simulink model "sampleModel238_pp_991_1"  (R2021b)
settings: Solver=VariableStepAuto  StartTime=0.0  StopTime=10.0  RelTol=1e-3
undefined symbols (not defined in the file): DiscIntNeverNeededParam, Newton, Raphson
libraries: simulink x40, slpidlib x5
settings Model: Creator=user  LastModifiedBy=cemery

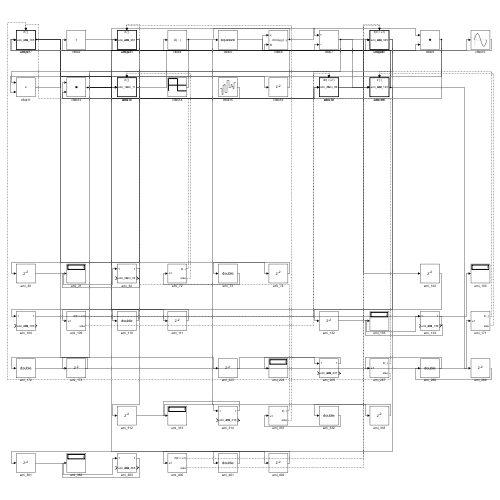
[thumbnail: Simulink's stored preview of the top-level diagram]
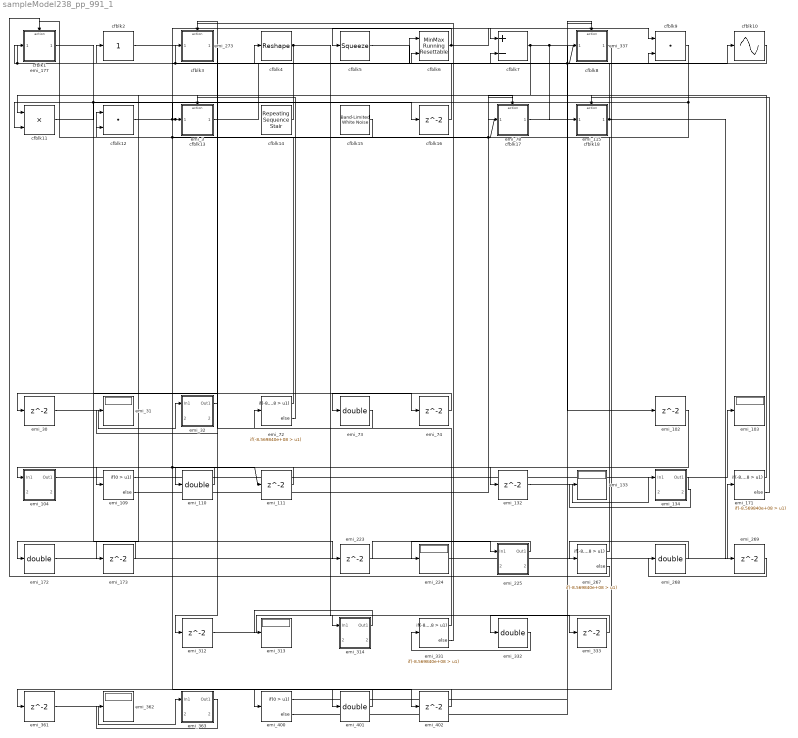
== system sampleModel238_pp_991_1 ==
  cfblk1 : Subsystem  TreatAsAtomicUnit=on
  cfblk10 : Sin  TimeSource=Use external signal  SampleTime=0
  cfblk11 : Product
  cfblk12 : DotProduct  InputSameDT=on  OutDataTypeStr=Inherit: Inherit via internal rule
  cfblk13 : Subsystem  TreatAsAtomicUnit=on
  cfblk14 : simulink/Sources/Repeating Sequence Stair  OutValues=[504987243.712228, -428491998.363153]  tsamp=-1  OutMin=[]  OutMax=[]  OutDataTypeStr=double  OutputDataTypeScalingMode=double  OutDataType=fixdt(0,8)  ConRadixGroup=Best Precision: Vector-wise  OutScaling=2^-12
  cfblk15 : simulink/Sources/Band-Limited White Noise  Cov=[8048045641.743666]  Ts=0.1  seed=[4340023928.000000]
  cfblk16 : Delay  SampleTime=1
  cfblk17 : Subsystem  TreatAsAtomicUnit=on
  cfblk18 : Subsystem  TreatAsAtomicUnit=on
  cfblk2 : simulink/Math Operations/Slider Gain  gain=1  low=0  high=2
  cfblk3 : Subsystem  TreatAsAtomicUnit=on
  cfblk4 : Reshape
  cfblk5 : Squeeze
  cfblk6 : simulink/Math Operations/MinMax Running Resettable  Function=min  vinit=0.0
  cfblk7 : Sum  Inputs=+-
  cfblk8 : Subsystem  TreatAsAtomicUnit=on
  cfblk9 : DotProduct  InputSameDT=on  OutDataTypeStr=Inherit: Inherit via internal rule
  emi_{30,102,132,361} (4 alike) : Delay  SampleTime=1
  emi_{31,103,133,224,313,362} (6 alike) : Display
  emi_104 : Subsystem
  emi_109 : If  IfExpression=0 > u1  SampleTime=1
  emi_{73,110,172,268,332,401} (6 alike) : DataTypeConversion  OutDataTypeStr=double
  emi_111 : Delay  InitialCondition=0
  emi_115 : Subsystem  TreatAsAtomicUnit=on
  emi_134 : Subsystem
  emi_171 : If  IfExpression=-8.569840e+08 > u1  SampleTime=1
  emi_{74,173,269,333} (4 alike) : Delay  InitialCondition=-428491998.3632
  emi_177 : Subsystem  TreatAsAtomicUnit=on
  emi_223 : Delay
  emi_225 : Subsystem
  emi_267 : If  IfExpression=-8.569840e+08 > u1
  emi_273 : Subsystem  TreatAsAtomicUnit=on
  emi_3 : Subsystem  TreatAsAtomicUnit=on
  emi_312 : Delay
  emi_314 : Subsystem
  emi_32 : Subsystem
  emi_331 : If  IfExpression=-8.569840e+08 > u1
  emi_337 : Subsystem  TreatAsAtomicUnit=on
  emi_363 : Subsystem
  emi_400 : If  IfExpression=0 > u1
  emi_402 : Delay  InitialCondition=0
  emi_72 : If  IfExpression=-8.569840e+08 > u1
  emi_78 : Subsystem  TreatAsAtomicUnit=on
  wires:
  cfblk14/1 -> cfblk4/1
  cfblk9/1 -> cfblk12/1, cfblk11/2
  cfblk15/1 -> cfblk12/2
  cfblk10/1 -> cfblk6/2
  cfblk2/1 -> cfblk7/1
  cfblk6/1 -> cfblk9/1, cfblk5/1
  cfblk12/1 -> emi_111/1, emi_402/1, cfblk17/1(emi_76), emi_78/1(emi_85), cfblk8/1(emi_335), emi_337/1(emi_344)
  cfblk5/1 -> cfblk7/2
  cfblk11/1 -> cfblk16/1
  cfblk16/1 -> cfblk6/1
  cfblk13/1(emi_2) -> cfblk10/1
  emi_3/1(emi_11) -> emi_30/1
  emi_30/1 -> emi_32/1(In1)
  emi_32/1(Out1) -> emi_31/1
  emi_72/2 -> cfblk13/Action
  emi_72/1 -> emi_3/Action
  emi_73/1 -> emi_72/1
  emi_74/1 -> emi_73/1
  cfblk17/1(emi_77) -> cfblk9/2
  emi_78/1(emi_86) -> emi_102/1
  emi_102/1 -> emi_104/1(In1)
  emi_104/1(Out1) -> emi_103/1
  emi_109/2 -> cfblk17/Action
  emi_109/1 -> emi_78/Action
  emi_110/1 -> emi_109/1
  emi_111/1 -> emi_110/1
  cfblk7/1 -> cfblk18/1(emi_113), emi_115/1(emi_122), emi_173/1
  emi_115/1(emi_123) -> emi_132/1
  emi_132/1 -> emi_134/1(In1)
  emi_134/1(Out1) -> emi_133/1
  emi_171/2 -> cfblk18/Action
  emi_171/1 -> emi_115/Action
  emi_172/1 -> emi_171/1
  emi_173/1 -> emi_172/1
  cfblk18/1(emi_114) -> cfblk1/1(emi_175), emi_177/1(emi_184), emi_269/1
  cfblk1/1(emi_176) -> emi_3/1(emi_10), cfblk13/1(emi_1), emi_74/1
  emi_177/1(emi_185) -> emi_223/1
  emi_223/1 -> emi_225/1(In1)
  emi_225/1(Out1) -> emi_224/1
  emi_267/2 -> cfblk1/Action
  emi_267/1 -> emi_177/Action
  emi_268/1 -> emi_267/1
  emi_269/1 -> emi_268/1
  cfblk4/1 -> cfblk3/1(emi_271), emi_273/1(emi_280), emi_333/1
  cfblk3/1(emi_272) -> cfblk2/1
  emi_273/1(emi_281) -> emi_312/1
  emi_312/1 -> emi_314/1(In1)
  emi_314/1(Out1) -> emi_313/1
  emi_331/2 -> cfblk3/Action
  emi_331/1 -> emi_273/Action
  emi_332/1 -> emi_331/1
  emi_333/1 -> emi_332/1
  cfblk8/1(emi_336) -> cfblk11/1
  emi_337/1(emi_345) -> emi_361/1
  emi_361/1 -> emi_363/1(In1)
  emi_363/1(Out1) -> emi_362/1
  emi_400/2 -> cfblk8/Action
  emi_400/1 -> emi_337/Action
  emi_401/1 -> emi_400/1
  emi_402/1 -> emi_401/1

== system sampleModel238_pp_991_1/cfblk1 ==
  emi_175 : Inport
  Action Port : ActionPort  ActionPortLabel=else
  cfblk1 : Sum  Inputs=+
  emi_176 : Outport
  wires:
  emi_175/1 -> cfblk1/1
  cfblk1/1 -> emi_176/1

== system sampleModel238_pp_991_1/cfblk13 ==
  emi_1 : Inport
  Action Port : ActionPort  ActionPortLabel=else
  cfblk13 : Sqrt  Operator=rSqrt  AlgorithmType=Newton-Raphson  SaturateOnIntegerOverflow=on
  emi_2 : Outport
  wires:
  emi_1/1 -> cfblk13/1
  cfblk13/1 -> emi_2/1

== system sampleModel238_pp_991_1/cfblk17 ==
  emi_76 : Inport
  Action Port : ActionPort  ActionPortLabel=else
  cfblk17 : Delay  SampleTime=1
  emi_77 : Outport
  wires:
  emi_76/1 -> cfblk17/1
  cfblk17/1 -> emi_77/1

== system sampleModel238_pp_991_1/cfblk18 ==
  emi_113 : Inport
  Action Port : ActionPort  ActionPortLabel=else
  cfblk18 : Delay  SampleTime=1
  emi_114 : Outport
  wires:
  emi_113/1 -> cfblk18/1
  cfblk18/1 -> emi_114/1

== system sampleModel238_pp_991_1/cfblk3 ==
  emi_271 : Inport
  Action Port : ActionPort  ActionPortLabel=else
  cfblk3 : PermuteDimensions
  emi_272 : Outport
  wires:
  emi_271/1 -> cfblk3/1
  cfblk3/1 -> emi_272/1

== system sampleModel238_pp_991_1/cfblk8 ==
  emi_335 : Inport
  Action Port : ActionPort  ActionPortLabel=else
  cfblk8 : Rounding
  emi_336 : Outport
  wires:
  emi_335/1 -> cfblk8/1
  cfblk8/1 -> emi_336/1

== system sampleModel238_pp_991_1/emi_104 ==
  In1 : Inport
  emi_105 : Inport  Port=2
  emi_107 : Rounding
  emi_108 : Constant
  Out1 : Outport
  emi_106 : Outport  Port=2
  wires:
  In1/1 -> Out1/1
  emi_108/1 -> emi_107/1
  emi_107/1 -> emi_106/1

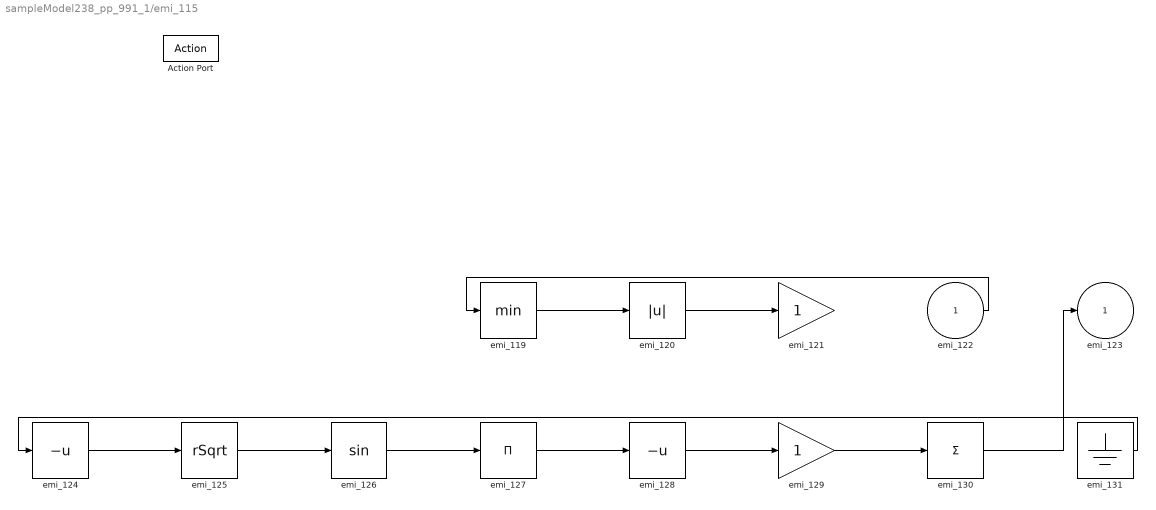
== system sampleModel238_pp_991_1/emi_115 ==
  emi_122 : Inport
  Action Port : ActionPort  ActionPortLabel=if(-8.569840e+08 > u1)
  emi_119 : MinMax  SampleTime=1
  emi_120 : Abs  SampleTime=1
  emi_121 : Gain  SampleTime=1
  emi_124 : UnaryMinus
  emi_125 : Sqrt  Operator=rSqrt  SaturateOnIntegerOverflow=on
  emi_126 : Trigonometry
  emi_127 : Product  Inputs=*
  emi_128 : UnaryMinus
  emi_129 : Gain
  emi_130 : Sum  Inputs=+
  emi_131 : Ground
  emi_123 : Outport
  wires:
  emi_122/1 -> emi_119/1
  emi_119/1 -> emi_120/1
  emi_120/1 -> emi_121/1
  emi_124/1 -> emi_125/1
  emi_125/1 -> emi_126/1
  emi_126/1 -> emi_127/1
  emi_127/1 -> emi_128/1
  emi_128/1 -> emi_129/1
  emi_129/1 -> emi_130/1
  emi_131/1 -> emi_124/1
  emi_130/1 -> emi_123/1

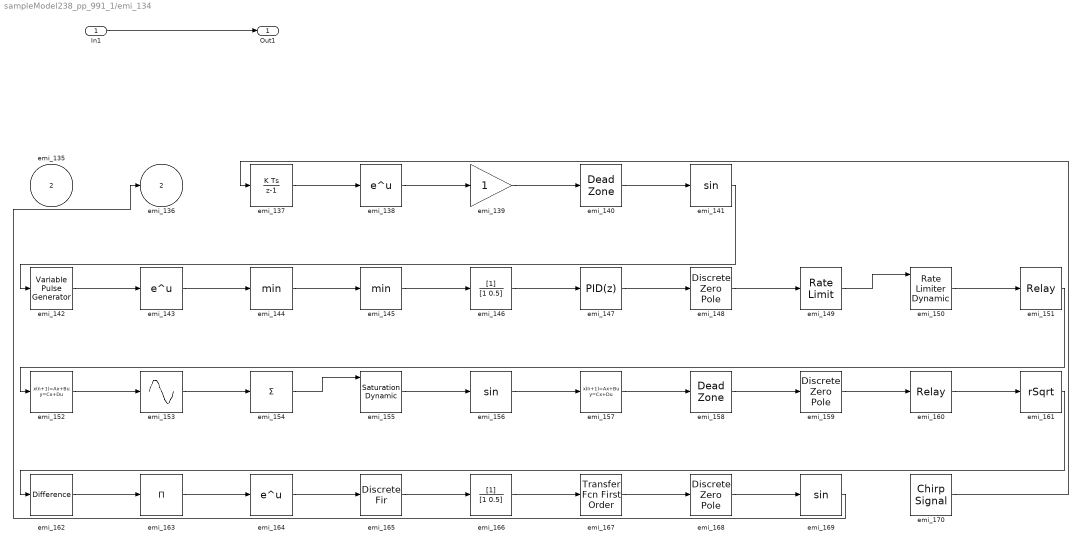
== system sampleModel238_pp_991_1/emi_134 ==
  In1 : Inport
  emi_135 : Inport  Port=2
  emi_137 : DiscreteIntegrator  SampleTime=-1  ICPrevOutput=DiscIntNeverNeededParam  ICPrevScaledInput=DiscIntNeverNeededParam
  emi_138 : Math  SaturateOnIntegerOverflow=on
  emi_139 : Gain
  emi_140 : DeadZone  SaturateOnIntegerOverflow=on
  emi_141 : Trigonometry
  emi_142 : VariablePulseGenerator  SampleTime=0.1
  emi_143 : Math  SaturateOnIntegerOverflow=on
  emi_144 : MinMax
  emi_145 : MinMax
  emi_146 : DiscreteFilter
  emi_147 : slpidlib/PID Controller  Controller=PID  Form=Parallel  TimeDomain=Discrete-time  UseExternalTs=off  SampleTime=-1  IntegratorMethod=Forward Euler  FilterMethod=Forward Euler  ControllerParametersSource=internal  P=1  I=1  D=0  UseFilter=on  N=100  TunerSelectOption=Transfer Function Based (PID Tuner App)  InitialConditionSource=internal  InitialConditionForIntegrator=0  InitialConditionForFilter=0  DifferentiatorICPrevScaledInput=0  ExternalReset=none  TrackingMode=off  Kt=1  LimitOutput=off  SatLimitsSource=internal  UpperSaturationLimit=inf  LowerSaturationLimit=-inf  LinearizeAsGain=off  AntiWindupMode=none  Kb=1  POutMin=[]  POutMax=[]  IOutMin=[]  IOutMax=[]  DOutMin=[]  DOutMax=[]  NOutMin=[]  NOutMax=[]  SumOutMin=[]  SumOutMax=[]  SaturationOutMin=[]  SaturationOutMax=[]  PParamMin=[]  PParamMax=[]  IParamMin=[]  IParamMax=[]  DParamMin=[]  DParamMax=[]  NParamMin=[]  NParamMax=[]  KbParamMin=[]  KbParamMax=[]  KtParamMin=[]  KtParamMax=[]  KbOutMin=[]  KbOutMax=[]  KtOutMin=[]  KtOutMax=[]  IntegratorOutMin=[]  IntegratorOutMax=[]  FilterOutMin=[]  FilterOutMax=[]  SumI1OutMin=[]  SumI1OutMax=[]  SumI2OutMin=[]  SumI2OutMax=[]  SumI3OutMin=[]  SumI3OutMax=[]  SumI4OutMin=[]  SumI4OutMax=[]  SumDOutMin=[]  SumDOutMax=[]  DifferentiatorOutMin=[]  DifferentiatorOutMax=[]  FilterDiffOutCoefMin=[]  FilterDiffOutCoefMax=[]  ReciprocalOutMin=[]  ReciprocalOutMax=[]  SumDenOutMin=[]  SumDenOutMax=[]  SumNumOutMin=[]  SumNumOutMax=[]  DivideOutMin=[]  DivideOutMax=[]  UdiffTsProdOutMin=[]  UdiffTsProdOutMax=[]  NTsProdOutMin=[]  NTsProdOutMax=[]  UintegralTsProdOutMin=[]  UintegralTsProdOutMax=[]  UngainTsProdOutMin=[]  UngainTsProdOutMax=[]  IntegratorContinuousStateAttributes=''  IntegratorStateMustResolveToSignalObject=off  IntegratorRTWStateStorageClass=Auto  FilterContinuousStateAttributes=''  FilterStateMustResolveToSignalObject=off  FilterRTWStateStorageClass=Auto  ParallelPVariant=InternalParameters  IdealPVariant=Disabled  IVariant=InternalParameters  DVariant=InternalParameters  IntegratorVariant=Discrete  SatVariant=Disabled  AWVariant=Passthrough  PCopyVariant=Disabled  TRVariant=Disabled  FdbkBlocksVariant=Forward  IdealPFdbkVariant=Disabled  SatFdbkVariant=Disabled  DerivativeFilterVariant=ForwardEulerFilter  NVariant=InternalParameters  NCopyVariant=Disabled  FilterICVariant=InternalICsFilter  IntegratorICVariant=InternalICs  ExternalResetVariant=Disabled  TRSumVariant=Passthrough  SumFdbkVariant=Disabled  SumVariant=Sum_PID  TsampFilterVariant=InternalTs  TsampNgainVariant=Passthrough  TsampIntegralVariant=Passthrough  ExternalSaturationOutDataTypeStr=Inherit: Same as second input
  emi_148 : DiscreteZeroPole  Poles=[0 0.5]  Gain=1  SampleTime=-1
  emi_149 : RateLimiter  SampleTimeMode=inherited
  emi_150 : simulink/Discontinuities/Rate Limiter Dynamic
  emi_151 : Relay
  emi_152 : DiscreteStateSpace  SampleTime=-1
  emi_153 : Sin  TimeSource=Use external signal  SampleTime=0
  emi_154 : Sum  Inputs=+
  emi_155 : simulink/Discontinuities/Saturation Dynamic  OutMin=[]  OutMax=[]  OutDataTypeStr=Inherit: Same as second input  OutDataType=fixdt(1, 16)  OutScaling=2^-10  DoSatur=off
  emi_156 : Trigonometry
  emi_157 : DiscreteStateSpace  SampleTime=-1
  emi_158 : DeadZone  SaturateOnIntegerOverflow=on
  emi_159 : DiscreteZeroPole  Poles=[0 0.5]  Gain=1  SampleTime=-1
  emi_160 : Relay
  emi_161 : Sqrt  Operator=rSqrt  SaturateOnIntegerOverflow=on
  emi_162 : simulink/Discrete/Difference  ICPrevInput=0.0  OutMin=[]  OutMax=[]  OutDataType=fixdt(1, 16)  OutScaling=2^-10  DoSatur=off
  emi_163 : Product  Inputs=*
  emi_164 : Math  SaturateOnIntegerOverflow=on
  emi_165 : DiscreteFir
  emi_166 : DiscreteFilter
  emi_167 : simulink/Discrete/Transfer Fcn First Order  PoleZ=0.95  ICPrevOutput=0.0  DoSatur=off
  emi_168 : DiscreteZeroPole  Poles=[0 0.5]  Gain=1  SampleTime=-1
  emi_169 : Trigonometry
  emi_170 : simulink/Sources/Chirp Signal  f1=0.1  T=100  f2=1
  Out1 : Outport
  emi_136 : Outport  Port=2
  wires:
  In1/1 -> Out1/1
  emi_137/1 -> emi_138/1
  emi_138/1 -> emi_139/1
  emi_139/1 -> emi_140/1
  emi_140/1 -> emi_141/1
  emi_141/1 -> emi_142/1
  emi_142/1 -> emi_143/1
  emi_143/1 -> emi_144/1
  emi_144/1 -> emi_145/1
  emi_145/1 -> emi_146/1
  emi_146/1 -> emi_147/1
  emi_147/1 -> emi_148/1
  emi_148/1 -> emi_149/1
  emi_149/1 -> emi_150/1
  emi_150/1 -> emi_151/1
  emi_151/1 -> emi_152/1
  emi_152/1 -> emi_153/1
  emi_153/1 -> emi_154/1
  emi_154/1 -> emi_155/1
  emi_155/1 -> emi_156/1
  emi_156/1 -> emi_157/1
  emi_157/1 -> emi_158/1
  emi_158/1 -> emi_159/1
  emi_159/1 -> emi_160/1
  emi_160/1 -> emi_161/1
  emi_161/1 -> emi_162/1
  emi_162/1 -> emi_163/1
  emi_163/1 -> emi_164/1
  emi_164/1 -> emi_165/1
  emi_165/1 -> emi_166/1
  emi_166/1 -> emi_167/1
  emi_167/1 -> emi_168/1
  emi_168/1 -> emi_169/1
  emi_170/1 -> emi_137/1
  emi_169/1 -> emi_136/1

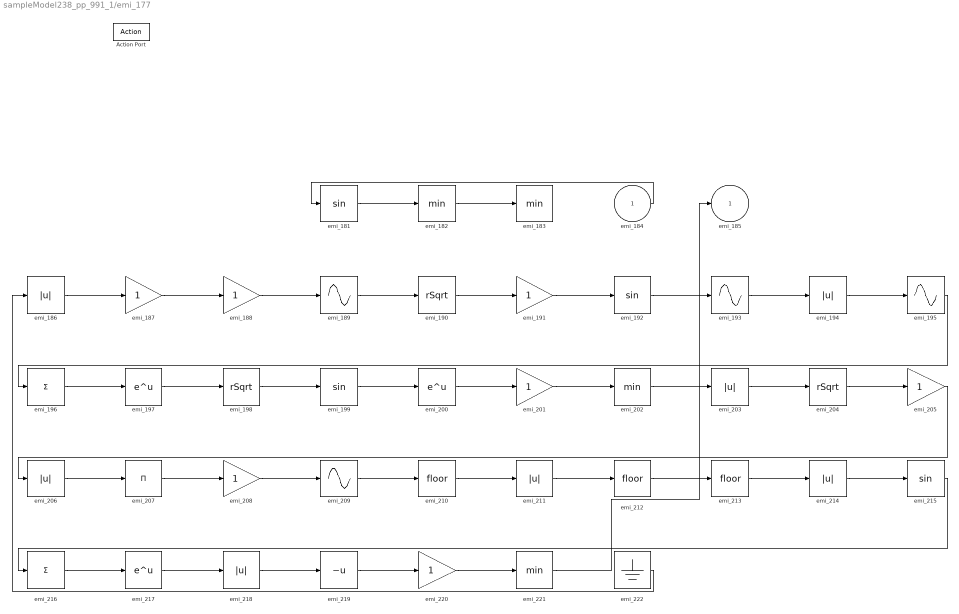
== system sampleModel238_pp_991_1/emi_177 ==
  emi_184 : Inport
  Action Port : ActionPort  ActionPortLabel=if(-8.569840e+08 > u1)
  emi_{181,192,199,215} (4 alike) : Trigonometry
  emi_{182..183,202,221} (4 alike) : MinMax
  emi_{186,194,203,206,211,214,218} (7 alike) : Abs
  emi_{187..188,191,201,205,208,220} (7 alike) : Gain
  emi_{189,193,195,209} (4 alike) : Sin  TimeSource=Use external signal  SampleTime=0
  emi_190 : Sqrt  Operator=rSqrt  SaturateOnIntegerOverflow=on
  emi_196 : Sum  Inputs=+
  emi_197 : Math  SaturateOnIntegerOverflow=on
  emi_198 : Sqrt  Operator=rSqrt  SaturateOnIntegerOverflow=on
  emi_200 : Math  SaturateOnIntegerOverflow=on
  emi_204 : Sqrt  Operator=rSqrt  SaturateOnIntegerOverflow=on
  emi_207 : Product  Inputs=*
  emi_210 : Rounding
  emi_212 : Rounding
  emi_213 : Rounding
  emi_216 : Sum  Inputs=+
  emi_217 : Math  SaturateOnIntegerOverflow=on
  emi_219 : UnaryMinus
  emi_222 : Ground
  emi_185 : Outport
  wires:
  emi_184/1 -> emi_181/1
  emi_181/1 -> emi_182/1
  emi_182/1 -> emi_183/1
  emi_186/1 -> emi_187/1
  emi_187/1 -> emi_188/1
  emi_188/1 -> emi_189/1
  emi_189/1 -> emi_190/1
  emi_190/1 -> emi_191/1
  emi_191/1 -> emi_192/1
  emi_192/1 -> emi_193/1
  emi_193/1 -> emi_194/1
  emi_194/1 -> emi_195/1
  emi_195/1 -> emi_196/1
  emi_196/1 -> emi_197/1
  emi_197/1 -> emi_198/1
  emi_198/1 -> emi_199/1
  emi_199/1 -> emi_200/1
  emi_200/1 -> emi_201/1
  emi_201/1 -> emi_202/1
  emi_202/1 -> emi_203/1
  emi_203/1 -> emi_204/1
  emi_204/1 -> emi_205/1
  emi_205/1 -> emi_206/1
  emi_206/1 -> emi_207/1
  emi_207/1 -> emi_208/1
  emi_208/1 -> emi_209/1
  emi_209/1 -> emi_210/1
  emi_210/1 -> emi_211/1
  emi_211/1 -> emi_212/1
  emi_212/1 -> emi_213/1
  emi_213/1 -> emi_214/1
  emi_214/1 -> emi_215/1
  emi_215/1 -> emi_216/1
  emi_216/1 -> emi_217/1
  emi_217/1 -> emi_218/1
  emi_218/1 -> emi_219/1
  emi_219/1 -> emi_220/1
  emi_220/1 -> emi_221/1
  emi_222/1 -> emi_186/1
  emi_221/1 -> emi_185/1

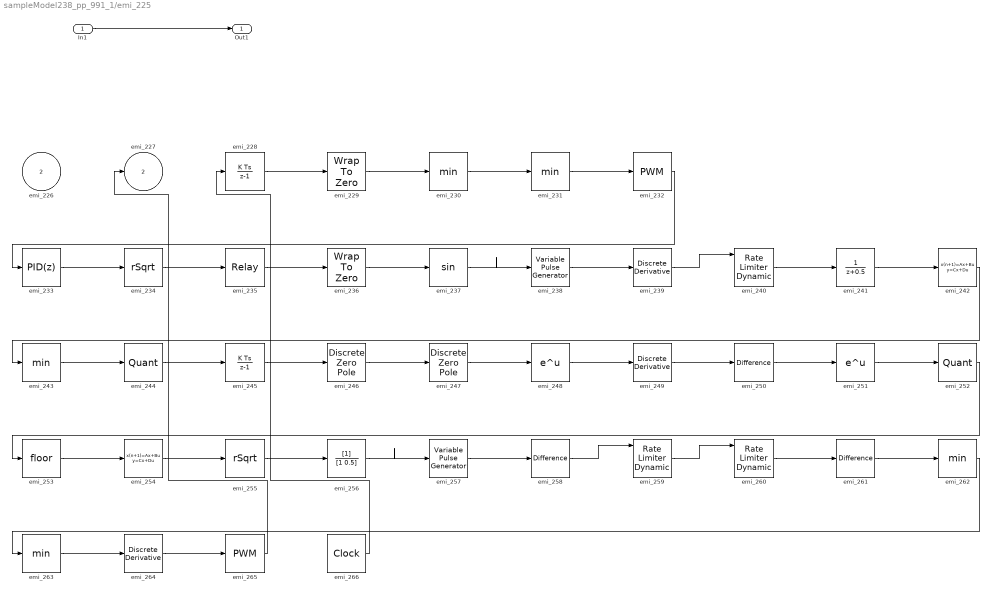
== system sampleModel238_pp_991_1/emi_225 ==
  In1 : Inport
  emi_226 : Inport  Port=2
  emi_228 : DiscreteIntegrator  SampleTime=-1  ICPrevOutput=DiscIntNeverNeededParam  ICPrevScaledInput=DiscIntNeverNeededParam
  emi_229 : simulink/Discontinuities/Wrap To Zero  Threshold=255
      settings: SourceProductBaseCode=SL
  emi_{230..231,243,262..263} (5 alike) : MinMax
  emi_232 : simulink/Discontinuities/PWM  DisableCoverage=on  Period=1  DisallowZeroDutyCycle=off  RunAtFixedTimeIntervals=off  SampleTime=0.1
  emi_233 : slpidlib/PID Controller  Controller=PID  Form=Parallel  TimeDomain=Discrete-time  UseExternalTs=off  SampleTime=-1  IntegratorMethod=Forward Euler  FilterMethod=Forward Euler  ControllerParametersSource=internal  P=1  I=1  D=0  UseFilter=on  N=100  TunerSelectOption=Transfer Function Based (PID Tuner App)  InitialConditionSource=internal  InitialConditionForIntegrator=0  InitialConditionForFilter=0  DifferentiatorICPrevScaledInput=0  ExternalReset=none  TrackingMode=off  Kt=1  LimitOutput=off  SatLimitsSource=internal  UpperSaturationLimit=inf  LowerSaturationLimit=-inf  LinearizeAsGain=off  AntiWindupMode=none  Kb=1  POutMin=[]  POutMax=[]  IOutMin=[]  IOutMax=[]  DOutMin=[]  DOutMax=[]  NOutMin=[]  NOutMax=[]  SumOutMin=[]  SumOutMax=[]  SaturationOutMin=[]  SaturationOutMax=[]  PParamMin=[]  PParamMax=[]  IParamMin=[]  IParamMax=[]  DParamMin=[]  DParamMax=[]  NParamMin=[]  NParamMax=[]  KbParamMin=[]  KbParamMax=[]  KtParamMin=[]  KtParamMax=[]  KbOutMin=[]  KbOutMax=[]  KtOutMin=[]  KtOutMax=[]  IntegratorOutMin=[]  IntegratorOutMax=[]  FilterOutMin=[]  FilterOutMax=[]  SumI1OutMin=[]  SumI1OutMax=[]  SumI2OutMin=[]  SumI2OutMax=[]  SumI3OutMin=[]  SumI3OutMax=[]  SumI4OutMin=[]  SumI4OutMax=[]  SumDOutMin=[]  SumDOutMax=[]  DifferentiatorOutMin=[]  DifferentiatorOutMax=[]  FilterDiffOutCoefMin=[]  FilterDiffOutCoefMax=[]  ReciprocalOutMin=[]  ReciprocalOutMax=[]  SumDenOutMin=[]  SumDenOutMax=[]  SumNumOutMin=[]  SumNumOutMax=[]  DivideOutMin=[]  DivideOutMax=[]  UdiffTsProdOutMin=[]  UdiffTsProdOutMax=[]  NTsProdOutMin=[]  NTsProdOutMax=[]  UintegralTsProdOutMin=[]  UintegralTsProdOutMax=[]  UngainTsProdOutMin=[]  UngainTsProdOutMax=[]  IntegratorContinuousStateAttributes=''  IntegratorStateMustResolveToSignalObject=off  IntegratorRTWStateStorageClass=Auto  FilterContinuousStateAttributes=''  FilterStateMustResolveToSignalObject=off  FilterRTWStateStorageClass=Auto  ParallelPVariant=InternalParameters  IdealPVariant=Disabled  IVariant=InternalParameters  DVariant=InternalParameters  IntegratorVariant=Discrete  SatVariant=Disabled  AWVariant=Passthrough  PCopyVariant=Disabled  TRVariant=Disabled  FdbkBlocksVariant=Forward  IdealPFdbkVariant=Disabled  SatFdbkVariant=Disabled  DerivativeFilterVariant=ForwardEulerFilter  NVariant=InternalParameters  NCopyVariant=Disabled  FilterICVariant=InternalICsFilter  IntegratorICVariant=InternalICs  ExternalResetVariant=Disabled  TRSumVariant=Passthrough  SumFdbkVariant=Disabled  SumVariant=Sum_PID  TsampFilterVariant=InternalTs  TsampNgainVariant=Passthrough  TsampIntegralVariant=Passthrough  ExternalSaturationOutDataTypeStr=Inherit: Same as second input
  emi_234 : Sqrt  Operator=rSqrt  SaturateOnIntegerOverflow=on
  emi_235 : Relay
  emi_236 : simulink/Discontinuities/Wrap To Zero  Threshold=255
      settings: SourceProductBaseCode=SL
  emi_237 : Trigonometry
  emi_238 : VariablePulseGenerator  SampleTime=0.1
  emi_239 : simulink/Discrete/Discrete Derivative  gainval=1.0  ICPrevScaledInput=0.0  OutMin=[]  OutMax=[]  OutDataType=fixdt(1, 16)  OutScaling=2^-10  DoSatur=off
  emi_240 : simulink/Discontinuities/Rate Limiter Dynamic
  emi_241 : DiscreteTransferFcn
  emi_242 : DiscreteStateSpace  SampleTime=-1
  emi_244 : Quantizer
  emi_245 : DiscreteIntegrator  SampleTime=-1  ICPrevOutput=DiscIntNeverNeededParam  ICPrevScaledInput=DiscIntNeverNeededParam
  emi_246 : DiscreteZeroPole  Poles=[0 0.5]  Gain=1  SampleTime=-1
  emi_247 : DiscreteZeroPole  Poles=[0 0.5]  Gain=1  SampleTime=-1
  emi_248 : Math  SaturateOnIntegerOverflow=on
  emi_249 : simulink/Discrete/Discrete Derivative  gainval=1.0  ICPrevScaledInput=0.0  OutMin=[]  OutMax=[]  OutDataType=fixdt(1, 16)  OutScaling=2^-10  DoSatur=off
  emi_250 : simulink/Discrete/Difference  ICPrevInput=0.0  OutMin=[]  OutMax=[]  OutDataType=fixdt(1, 16)  OutScaling=2^-10  DoSatur=off
  emi_251 : Math  SaturateOnIntegerOverflow=on
  emi_252 : Quantizer
  emi_253 : Rounding
  emi_254 : DiscreteStateSpace  SampleTime=-1
  emi_255 : Sqrt  Operator=rSqrt  SaturateOnIntegerOverflow=on
  emi_256 : DiscreteFilter
  emi_257 : VariablePulseGenerator  SampleTime=0.1
  emi_258 : simulink/Discrete/Difference  ICPrevInput=0.0  OutMin=[]  OutMax=[]  OutDataType=fixdt(1, 16)  OutScaling=2^-10  DoSatur=off
  emi_259 : simulink/Discontinuities/Rate Limiter Dynamic
  emi_260 : simulink/Discontinuities/Rate Limiter Dynamic
  emi_261 : simulink/Discrete/Difference  ICPrevInput=0.0  OutMin=[]  OutMax=[]  OutDataType=fixdt(1, 16)  OutScaling=2^-10  DoSatur=off
  emi_264 : simulink/Discrete/Discrete Derivative  gainval=1.0  ICPrevScaledInput=0.0  OutMin=[]  OutMax=[]  OutDataType=fixdt(1, 16)  OutScaling=2^-10  DoSatur=off
  emi_265 : simulink/Discontinuities/PWM  DisableCoverage=on  Period=1  DisallowZeroDutyCycle=off  RunAtFixedTimeIntervals=off  SampleTime=0.1
  emi_266 : DigitalClock
  Out1 : Outport
  emi_227 : Outport  Port=2
  wires:
  In1/1 -> Out1/1
  emi_228/1 -> emi_229/1
  emi_229/1 -> emi_230/1
  emi_230/1 -> emi_231/1
  emi_231/1 -> emi_232/1
  emi_232/1 -> emi_233/1
  emi_233/1 -> emi_234/1
  emi_234/1 -> emi_235/1
  emi_235/1 -> emi_236/1
  emi_236/1 -> emi_237/1
  emi_237/1 -> emi_238/1
  emi_238/1 -> emi_239/1
  emi_239/1 -> emi_240/1
  emi_240/1 -> emi_241/1
  emi_241/1 -> emi_242/1
  emi_242/1 -> emi_243/1
  emi_243/1 -> emi_244/1
  emi_244/1 -> emi_245/1
  emi_245/1 -> emi_246/1
  emi_246/1 -> emi_247/1
  emi_247/1 -> emi_248/1
  emi_248/1 -> emi_249/1
  emi_249/1 -> emi_250/1
  emi_250/1 -> emi_251/1
  emi_251/1 -> emi_252/1
  emi_252/1 -> emi_253/1
  emi_253/1 -> emi_254/1
  emi_254/1 -> emi_255/1
  emi_255/1 -> emi_256/1
  emi_256/1 -> emi_257/1
  emi_257/1 -> emi_258/1
  emi_258/1 -> emi_259/1
  emi_259/1 -> emi_260/1
  emi_260/1 -> emi_261/1
  emi_261/1 -> emi_262/1
  emi_262/1 -> emi_263/1
  emi_263/1 -> emi_264/1
  emi_264/1 -> emi_265/1
  emi_266/1 -> emi_228/1
  emi_265/1 -> emi_227/1

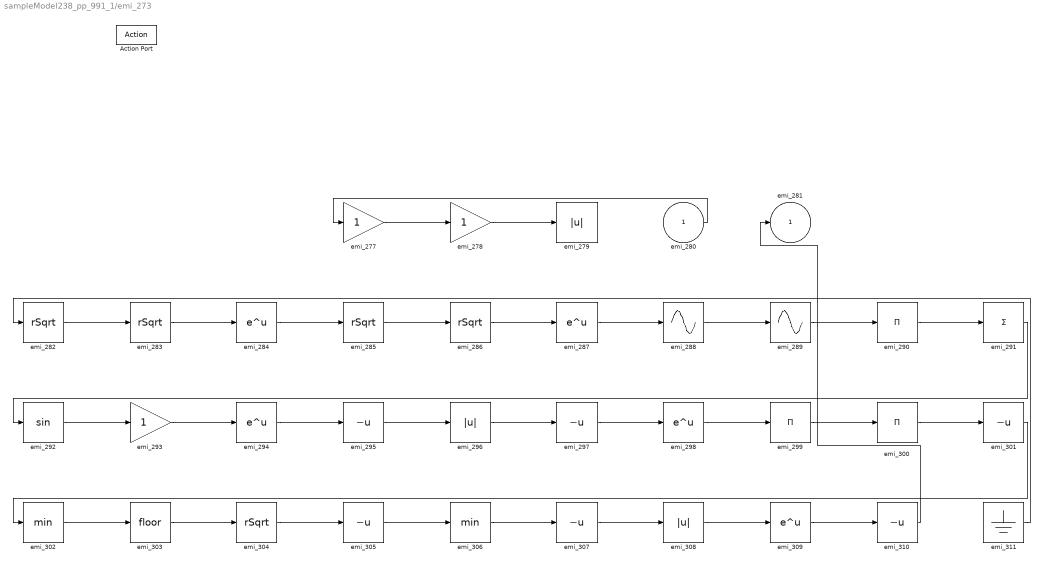
== system sampleModel238_pp_991_1/emi_273 ==
  emi_280 : Inport
  Action Port : ActionPort  ActionPortLabel=if(-8.569840e+08 > u1)
  emi_277 : Gain
  emi_278 : Gain
  emi_279 : Abs
  emi_{282..283,285..286,304} (5 alike) : Sqrt  Operator=rSqrt  SaturateOnIntegerOverflow=on
  emi_{284,287,294,298,309} (5 alike) : Math  SaturateOnIntegerOverflow=on
  emi_288 : Sin  TimeSource=Use external signal  SampleTime=0
  emi_289 : Sin  TimeSource=Use external signal  SampleTime=0
  emi_290 : Product  Inputs=*
  emi_291 : Sum  Inputs=+
  emi_292 : Trigonometry
  emi_293 : Gain
  emi_{295,297,301,305,307,310} (6 alike) : UnaryMinus
  emi_296 : Abs
  emi_299 : Product  Inputs=*
  emi_300 : Product  Inputs=*
  emi_302 : MinMax
  emi_303 : Rounding
  emi_306 : MinMax
  emi_308 : Abs
  emi_311 : Ground
  emi_281 : Outport
  wires:
  emi_280/1 -> emi_277/1
  emi_277/1 -> emi_278/1
  emi_278/1 -> emi_279/1
  emi_282/1 -> emi_283/1
  emi_283/1 -> emi_284/1
  emi_284/1 -> emi_285/1
  emi_285/1 -> emi_286/1
  emi_286/1 -> emi_287/1
  emi_287/1 -> emi_288/1
  emi_288/1 -> emi_289/1
  emi_289/1 -> emi_290/1
  emi_290/1 -> emi_291/1
  emi_291/1 -> emi_292/1
  emi_292/1 -> emi_293/1
  emi_293/1 -> emi_294/1
  emi_294/1 -> emi_295/1
  emi_295/1 -> emi_296/1
  emi_296/1 -> emi_297/1
  emi_297/1 -> emi_298/1
  emi_298/1 -> emi_299/1
  emi_299/1 -> emi_300/1
  emi_300/1 -> emi_301/1
  emi_301/1 -> emi_302/1
  emi_302/1 -> emi_303/1
  emi_303/1 -> emi_304/1
  emi_304/1 -> emi_305/1
  emi_305/1 -> emi_306/1
  emi_306/1 -> emi_307/1
  emi_307/1 -> emi_308/1
  emi_308/1 -> emi_309/1
  emi_309/1 -> emi_310/1
  emi_311/1 -> emi_282/1
  emi_310/1 -> emi_281/1

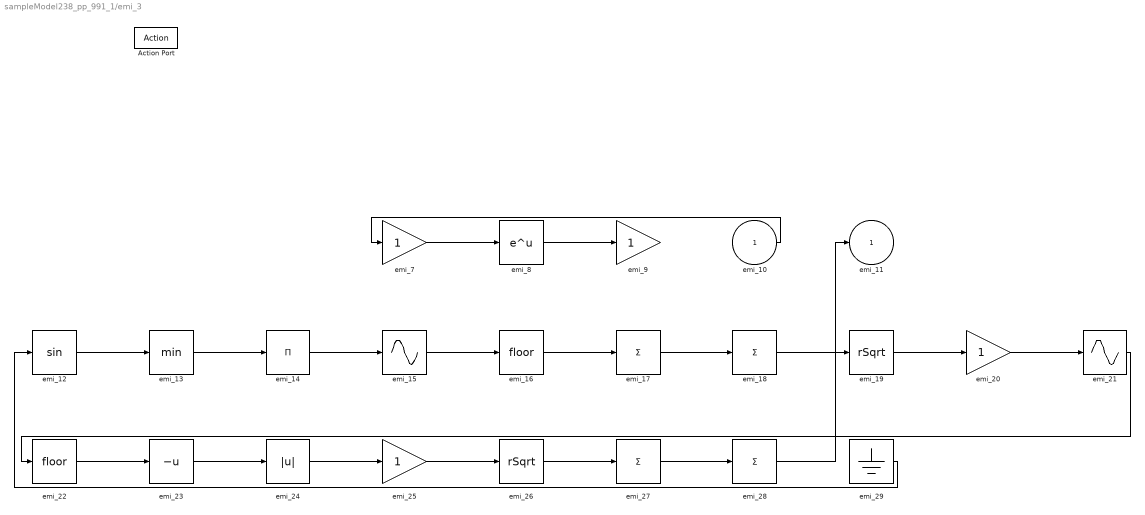
== system sampleModel238_pp_991_1/emi_3 ==
  emi_10 : Inport
  Action Port : ActionPort  ActionPortLabel=if(-8.569840e+08 > u1)
  emi_12 : Trigonometry
  emi_13 : MinMax
  emi_14 : Product  Inputs=*
  emi_15 : Sin  TimeSource=Use external signal  SampleTime=0
  emi_16 : Rounding
  emi_{17..18,27..28} (4 alike) : Sum  Inputs=+
  emi_19 : Sqrt  Operator=rSqrt  SaturateOnIntegerOverflow=on
  emi_{7,9,20,25} (4 alike) : Gain
  emi_21 : Sin  TimeSource=Use external signal  SampleTime=0
  emi_22 : Rounding
  emi_23 : UnaryMinus
  emi_24 : Abs
  emi_26 : Sqrt  Operator=rSqrt  SaturateOnIntegerOverflow=on
  emi_29 : Ground
  emi_8 : Math  SaturateOnIntegerOverflow=on
  emi_11 : Outport
  wires:
  emi_10/1 -> emi_7/1
  emi_7/1 -> emi_8/1
  emi_8/1 -> emi_9/1
  emi_12/1 -> emi_13/1
  emi_13/1 -> emi_14/1
  emi_14/1 -> emi_15/1
  emi_15/1 -> emi_16/1
  emi_16/1 -> emi_17/1
  emi_17/1 -> emi_18/1
  emi_18/1 -> emi_19/1
  emi_19/1 -> emi_20/1
  emi_20/1 -> emi_21/1
  emi_21/1 -> emi_22/1
  emi_22/1 -> emi_23/1
  emi_23/1 -> emi_24/1
  emi_24/1 -> emi_25/1
  emi_25/1 -> emi_26/1
  emi_26/1 -> emi_27/1
  emi_27/1 -> emi_28/1
  emi_29/1 -> emi_12/1
  emi_28/1 -> emi_11/1

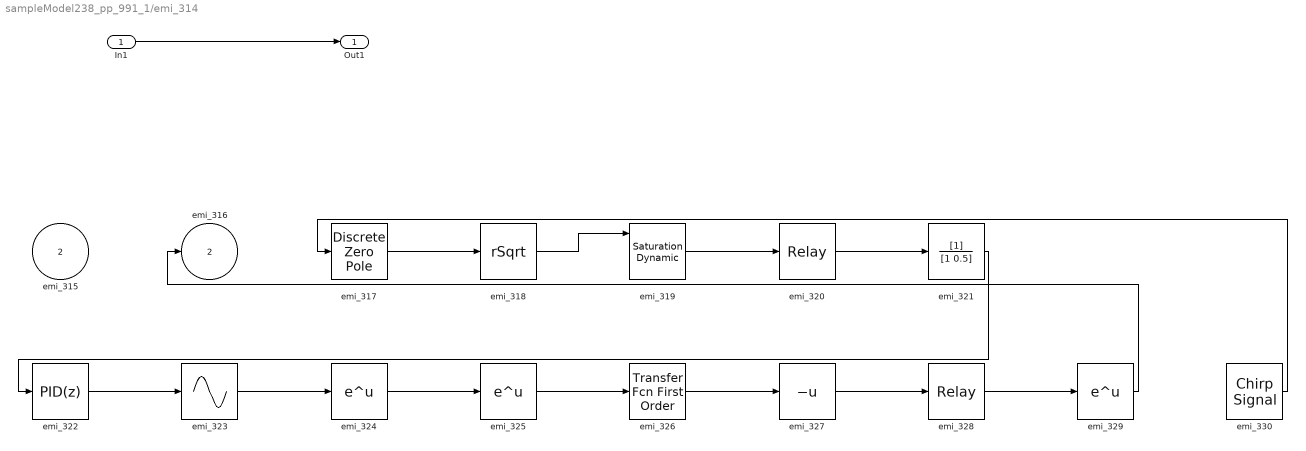
== system sampleModel238_pp_991_1/emi_314 ==
  In1 : Inport
  emi_315 : Inport  Port=2
  emi_317 : DiscreteZeroPole  Poles=[0 0.5]  Gain=1  SampleTime=-1
  emi_318 : Sqrt  Operator=rSqrt  SaturateOnIntegerOverflow=on
  emi_319 : simulink/Discontinuities/Saturation Dynamic  OutMin=[]  OutMax=[]  OutDataTypeStr=Inherit: Same as second input  OutDataType=fixdt(1, 16)  OutScaling=2^-10  DoSatur=off
  emi_320 : Relay
  emi_321 : DiscreteFilter
  emi_322 : slpidlib/PID Controller  Controller=PID  Form=Parallel  TimeDomain=Discrete-time  UseExternalTs=off  SampleTime=-1  IntegratorMethod=Forward Euler  FilterMethod=Forward Euler  ControllerParametersSource=internal  P=1  I=1  D=0  UseFilter=on  N=100  TunerSelectOption=Transfer Function Based (PID Tuner App)  InitialConditionSource=internal  InitialConditionForIntegrator=0  InitialConditionForFilter=0  DifferentiatorICPrevScaledInput=0  ExternalReset=none  TrackingMode=off  Kt=1  LimitOutput=off  SatLimitsSource=internal  UpperSaturationLimit=inf  LowerSaturationLimit=-inf  LinearizeAsGain=off  AntiWindupMode=none  Kb=1  POutMin=[]  POutMax=[]  IOutMin=[]  IOutMax=[]  DOutMin=[]  DOutMax=[]  NOutMin=[]  NOutMax=[]  SumOutMin=[]  SumOutMax=[]  SaturationOutMin=[]  SaturationOutMax=[]  PParamMin=[]  PParamMax=[]  IParamMin=[]  IParamMax=[]  DParamMin=[]  DParamMax=[]  NParamMin=[]  NParamMax=[]  KbParamMin=[]  KbParamMax=[]  KtParamMin=[]  KtParamMax=[]  KbOutMin=[]  KbOutMax=[]  KtOutMin=[]  KtOutMax=[]  IntegratorOutMin=[]  IntegratorOutMax=[]  FilterOutMin=[]  FilterOutMax=[]  SumI1OutMin=[]  SumI1OutMax=[]  SumI2OutMin=[]  SumI2OutMax=[]  SumI3OutMin=[]  SumI3OutMax=[]  SumI4OutMin=[]  SumI4OutMax=[]  SumDOutMin=[]  SumDOutMax=[]  DifferentiatorOutMin=[]  DifferentiatorOutMax=[]  FilterDiffOutCoefMin=[]  FilterDiffOutCoefMax=[]  ReciprocalOutMin=[]  ReciprocalOutMax=[]  SumDenOutMin=[]  SumDenOutMax=[]  SumNumOutMin=[]  SumNumOutMax=[]  DivideOutMin=[]  DivideOutMax=[]  UdiffTsProdOutMin=[]  UdiffTsProdOutMax=[]  NTsProdOutMin=[]  NTsProdOutMax=[]  UintegralTsProdOutMin=[]  UintegralTsProdOutMax=[]  UngainTsProdOutMin=[]  UngainTsProdOutMax=[]  IntegratorContinuousStateAttributes=''  IntegratorStateMustResolveToSignalObject=off  IntegratorRTWStateStorageClass=Auto  FilterContinuousStateAttributes=''  FilterStateMustResolveToSignalObject=off  FilterRTWStateStorageClass=Auto  ParallelPVariant=InternalParameters  IdealPVariant=Disabled  IVariant=InternalParameters  DVariant=InternalParameters  IntegratorVariant=Discrete  SatVariant=Disabled  AWVariant=Passthrough  PCopyVariant=Disabled  TRVariant=Disabled  FdbkBlocksVariant=Forward  IdealPFdbkVariant=Disabled  SatFdbkVariant=Disabled  DerivativeFilterVariant=ForwardEulerFilter  NVariant=InternalParameters  NCopyVariant=Disabled  FilterICVariant=InternalICsFilter  IntegratorICVariant=InternalICs  ExternalResetVariant=Disabled  TRSumVariant=Passthrough  SumFdbkVariant=Disabled  SumVariant=Sum_PID  TsampFilterVariant=InternalTs  TsampNgainVariant=Passthrough  TsampIntegralVariant=Passthrough  ExternalSaturationOutDataTypeStr=Inherit: Same as second input
  emi_323 : Sin  TimeSource=Use external signal  SampleTime=0
  emi_324 : Math  SaturateOnIntegerOverflow=on
  emi_325 : Math  SaturateOnIntegerOverflow=on
  emi_326 : simulink/Discrete/Transfer Fcn First Order  PoleZ=0.95  ICPrevOutput=0.0  DoSatur=off
  emi_327 : UnaryMinus
  emi_328 : Relay
  emi_329 : Math  SaturateOnIntegerOverflow=on
  emi_330 : simulink/Sources/Chirp Signal  f1=0.1  T=100  f2=1
  Out1 : Outport
  emi_316 : Outport  Port=2
  wires:
  In1/1 -> Out1/1
  emi_317/1 -> emi_318/1
  emi_318/1 -> emi_319/1
  emi_319/1 -> emi_320/1
  emi_320/1 -> emi_321/1
  emi_321/1 -> emi_322/1
  emi_322/1 -> emi_323/1
  emi_323/1 -> emi_324/1
  emi_324/1 -> emi_325/1
  emi_325/1 -> emi_326/1
  emi_326/1 -> emi_327/1
  emi_327/1 -> emi_328/1
  emi_328/1 -> emi_329/1
  emi_330/1 -> emi_317/1
  emi_329/1 -> emi_316/1

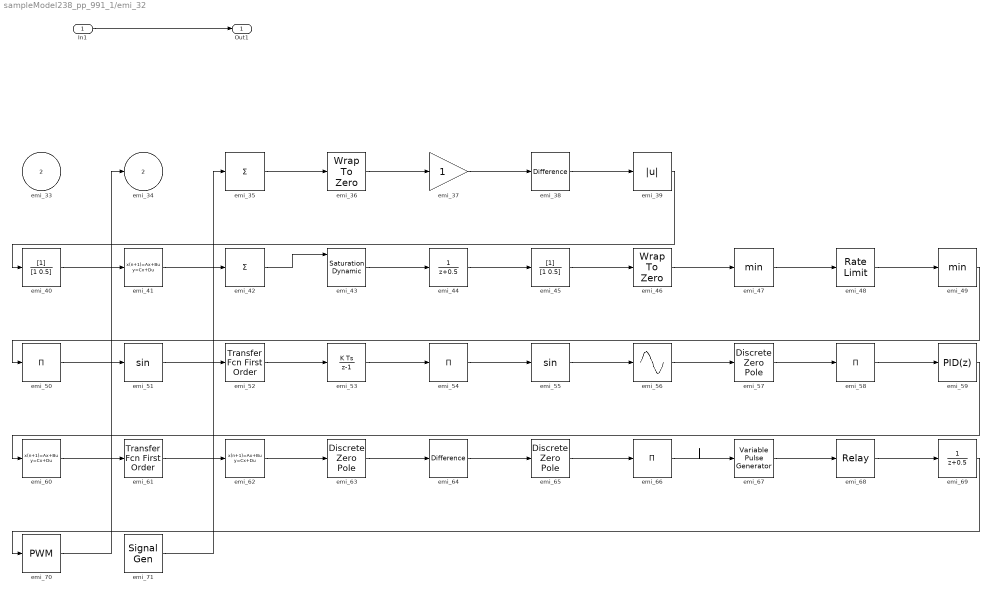
== system sampleModel238_pp_991_1/emi_32 ==
  In1 : Inport
  emi_33 : Inport  Port=2
  emi_35 : Sum  Inputs=+
  emi_36 : simulink/Discontinuities/Wrap To Zero  Threshold=255
      settings: SourceProductBaseCode=SL
  emi_37 : Gain
  emi_38 : simulink/Discrete/Difference  ICPrevInput=0.0  OutMin=[]  OutMax=[]  OutDataType=fixdt(1, 16)  OutScaling=2^-10  DoSatur=off
  emi_39 : Abs
  emi_40 : DiscreteFilter
  emi_41 : DiscreteStateSpace  SampleTime=-1
  emi_42 : Sum  Inputs=+
  emi_43 : simulink/Discontinuities/Saturation Dynamic  OutMin=[]  OutMax=[]  OutDataTypeStr=Inherit: Same as second input  OutDataType=fixdt(1, 16)  OutScaling=2^-10  DoSatur=off
  emi_44 : DiscreteTransferFcn
  emi_45 : DiscreteFilter
  emi_46 : simulink/Discontinuities/Wrap To Zero  Threshold=255
      settings: SourceProductBaseCode=SL
  emi_47 : MinMax
  emi_48 : RateLimiter  SampleTimeMode=inherited
  emi_49 : MinMax
  emi_{50,54,58,66} (4 alike) : Product  Inputs=*
  emi_51 : Trigonometry
  emi_52 : simulink/Discrete/Transfer Fcn First Order  PoleZ=0.95  ICPrevOutput=0.0  DoSatur=off
  emi_53 : DiscreteIntegrator  SampleTime=-1  ICPrevOutput=DiscIntNeverNeededParam  ICPrevScaledInput=DiscIntNeverNeededParam
  emi_55 : Trigonometry
  emi_56 : Sin  TimeSource=Use external signal  SampleTime=0
  emi_57 : DiscreteZeroPole  Poles=[0 0.5]  Gain=1  SampleTime=-1
  emi_59 : slpidlib/PID Controller  Controller=PID  Form=Parallel  TimeDomain=Discrete-time  UseExternalTs=off  SampleTime=-1  IntegratorMethod=Forward Euler  FilterMethod=Forward Euler  ControllerParametersSource=internal  P=1  I=1  D=0  UseFilter=on  N=100  TunerSelectOption=Transfer Function Based (PID Tuner App)  InitialConditionSource=internal  InitialConditionForIntegrator=0  InitialConditionForFilter=0  DifferentiatorICPrevScaledInput=0  ExternalReset=none  TrackingMode=off  Kt=1  LimitOutput=off  SatLimitsSource=internal  UpperSaturationLimit=inf  LowerSaturationLimit=-inf  LinearizeAsGain=off  AntiWindupMode=none  Kb=1  POutMin=[]  POutMax=[]  IOutMin=[]  IOutMax=[]  DOutMin=[]  DOutMax=[]  NOutMin=[]  NOutMax=[]  SumOutMin=[]  SumOutMax=[]  SaturationOutMin=[]  SaturationOutMax=[]  PParamMin=[]  PParamMax=[]  IParamMin=[]  IParamMax=[]  DParamMin=[]  DParamMax=[]  NParamMin=[]  NParamMax=[]  KbParamMin=[]  KbParamMax=[]  KtParamMin=[]  KtParamMax=[]  KbOutMin=[]  KbOutMax=[]  KtOutMin=[]  KtOutMax=[]  IntegratorOutMin=[]  IntegratorOutMax=[]  FilterOutMin=[]  FilterOutMax=[]  SumI1OutMin=[]  SumI1OutMax=[]  SumI2OutMin=[]  SumI2OutMax=[]  SumI3OutMin=[]  SumI3OutMax=[]  SumI4OutMin=[]  SumI4OutMax=[]  SumDOutMin=[]  SumDOutMax=[]  DifferentiatorOutMin=[]  DifferentiatorOutMax=[]  FilterDiffOutCoefMin=[]  FilterDiffOutCoefMax=[]  ReciprocalOutMin=[]  ReciprocalOutMax=[]  SumDenOutMin=[]  SumDenOutMax=[]  SumNumOutMin=[]  SumNumOutMax=[]  DivideOutMin=[]  DivideOutMax=[]  UdiffTsProdOutMin=[]  UdiffTsProdOutMax=[]  NTsProdOutMin=[]  NTsProdOutMax=[]  UintegralTsProdOutMin=[]  UintegralTsProdOutMax=[]  UngainTsProdOutMin=[]  UngainTsProdOutMax=[]  IntegratorContinuousStateAttributes=''  IntegratorStateMustResolveToSignalObject=off  IntegratorRTWStateStorageClass=Auto  FilterContinuousStateAttributes=''  FilterStateMustResolveToSignalObject=off  FilterRTWStateStorageClass=Auto  ParallelPVariant=InternalParameters  IdealPVariant=Disabled  IVariant=InternalParameters  DVariant=InternalParameters  IntegratorVariant=Discrete  SatVariant=Disabled  AWVariant=Passthrough  PCopyVariant=Disabled  TRVariant=Disabled  FdbkBlocksVariant=Forward  IdealPFdbkVariant=Disabled  SatFdbkVariant=Disabled  DerivativeFilterVariant=ForwardEulerFilter  NVariant=InternalParameters  NCopyVariant=Disabled  FilterICVariant=InternalICsFilter  IntegratorICVariant=InternalICs  ExternalResetVariant=Disabled  TRSumVariant=Passthrough  SumFdbkVariant=Disabled  SumVariant=Sum_PID  TsampFilterVariant=InternalTs  TsampNgainVariant=Passthrough  TsampIntegralVariant=Passthrough  ExternalSaturationOutDataTypeStr=Inherit: Same as second input
  emi_60 : DiscreteStateSpace  SampleTime=-1
  emi_61 : simulink/Discrete/Transfer Fcn First Order  PoleZ=0.95  ICPrevOutput=0.0  DoSatur=off
  emi_62 : DiscreteStateSpace  SampleTime=-1
  emi_63 : DiscreteZeroPole  Poles=[0 0.5]  Gain=1  SampleTime=-1
  emi_64 : simulink/Discrete/Difference  ICPrevInput=0.0  OutMin=[]  OutMax=[]  OutDataType=fixdt(1, 16)  OutScaling=2^-10  DoSatur=off
  emi_65 : DiscreteZeroPole  Poles=[0 0.5]  Gain=1  SampleTime=-1
  emi_67 : VariablePulseGenerator  SampleTime=0.1
  emi_68 : Relay
  emi_69 : DiscreteTransferFcn
  emi_70 : simulink/Discontinuities/PWM  DisableCoverage=on  Period=1  DisallowZeroDutyCycle=off  RunAtFixedTimeIntervals=off  SampleTime=0.1
  emi_71 : SignalGenerator  Units=rad/sec
  Out1 : Outport
  emi_34 : Outport  Port=2
  wires:
  In1/1 -> Out1/1
  emi_35/1 -> emi_36/1
  emi_36/1 -> emi_37/1
  emi_37/1 -> emi_38/1
  emi_38/1 -> emi_39/1
  emi_39/1 -> emi_40/1
  emi_40/1 -> emi_41/1
  emi_41/1 -> emi_42/1
  emi_42/1 -> emi_43/1
  emi_43/1 -> emi_44/1
  emi_44/1 -> emi_45/1
  emi_45/1 -> emi_46/1
  emi_46/1 -> emi_47/1
  emi_47/1 -> emi_48/1
  emi_48/1 -> emi_49/1
  emi_49/1 -> emi_50/1
  emi_50/1 -> emi_51/1
  emi_51/1 -> emi_52/1
  emi_52/1 -> emi_53/1
  emi_53/1 -> emi_54/1
  emi_54/1 -> emi_55/1
  emi_55/1 -> emi_56/1
  emi_56/1 -> emi_57/1
  emi_57/1 -> emi_58/1
  emi_58/1 -> emi_59/1
  emi_59/1 -> emi_60/1
  emi_60/1 -> emi_61/1
  emi_61/1 -> emi_62/1
  emi_62/1 -> emi_63/1
  emi_63/1 -> emi_64/1
  emi_64/1 -> emi_65/1
  emi_65/1 -> emi_66/1
  emi_66/1 -> emi_67/1
  emi_67/1 -> emi_68/1
  emi_68/1 -> emi_69/1
  emi_69/1 -> emi_70/1
  emi_71/1 -> emi_35/1
  emi_70/1 -> emi_34/1

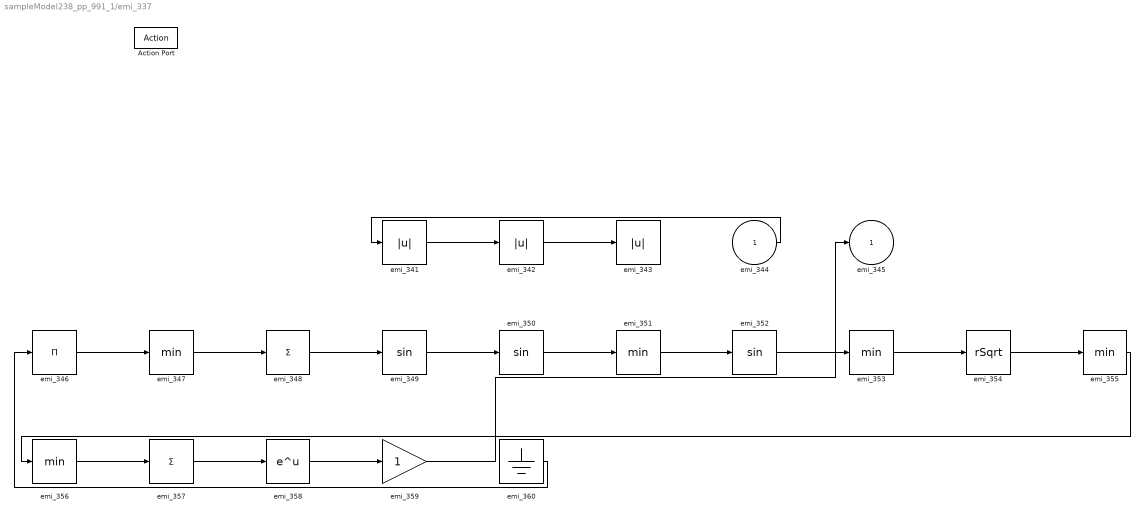
== system sampleModel238_pp_991_1/emi_337 ==
  emi_344 : Inport
  Action Port : ActionPort  ActionPortLabel=if(0 > u1)
  emi_341 : Abs
  emi_342 : Abs
  emi_343 : Abs
  emi_346 : Product  Inputs=*
  emi_{347,351,353,355..356} (5 alike) : MinMax
  emi_348 : Sum  Inputs=+
  emi_349 : Trigonometry
  emi_350 : Trigonometry
  emi_352 : Trigonometry
  emi_354 : Sqrt  Operator=rSqrt  SaturateOnIntegerOverflow=on
  emi_357 : Sum  Inputs=+
  emi_358 : Math  SaturateOnIntegerOverflow=on
  emi_359 : Gain
  emi_360 : Ground
  emi_345 : Outport
  wires:
  emi_344/1 -> emi_341/1
  emi_341/1 -> emi_342/1
  emi_342/1 -> emi_343/1
  emi_346/1 -> emi_347/1
  emi_347/1 -> emi_348/1
  emi_348/1 -> emi_349/1
  emi_349/1 -> emi_350/1
  emi_350/1 -> emi_351/1
  emi_351/1 -> emi_352/1
  emi_352/1 -> emi_353/1
  emi_353/1 -> emi_354/1
  emi_354/1 -> emi_355/1
  emi_355/1 -> emi_356/1
  emi_356/1 -> emi_357/1
  emi_357/1 -> emi_358/1
  emi_358/1 -> emi_359/1
  emi_360/1 -> emi_346/1
  emi_359/1 -> emi_345/1

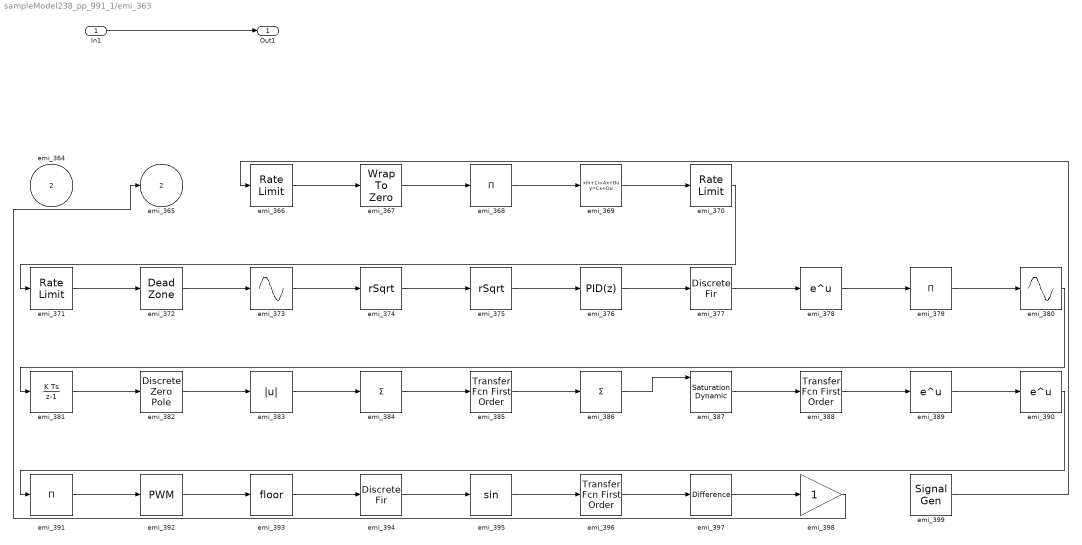
== system sampleModel238_pp_991_1/emi_363 ==
  In1 : Inport
  emi_364 : Inport  Port=2
  emi_366 : RateLimiter  SampleTimeMode=inherited
  emi_367 : simulink/Discontinuities/Wrap To Zero  Threshold=255
      settings: SourceProductBaseCode=SL
  emi_368 : Product  Inputs=*
  emi_369 : DiscreteStateSpace  SampleTime=-1
  emi_370 : RateLimiter  SampleTimeMode=inherited
  emi_371 : RateLimiter  SampleTimeMode=inherited
  emi_372 : DeadZone  SaturateOnIntegerOverflow=on
  emi_373 : Sin  TimeSource=Use external signal  SampleTime=0
  emi_374 : Sqrt  Operator=rSqrt  SaturateOnIntegerOverflow=on
  emi_375 : Sqrt  Operator=rSqrt  SaturateOnIntegerOverflow=on
  emi_376 : slpidlib/PID Controller  Controller=PID  Form=Parallel  TimeDomain=Discrete-time  UseExternalTs=off  SampleTime=-1  IntegratorMethod=Forward Euler  FilterMethod=Forward Euler  ControllerParametersSource=internal  P=1  I=1  D=0  UseFilter=on  N=100  TunerSelectOption=Transfer Function Based (PID Tuner App)  InitialConditionSource=internal  InitialConditionForIntegrator=0  InitialConditionForFilter=0  DifferentiatorICPrevScaledInput=0  ExternalReset=none  TrackingMode=off  Kt=1  LimitOutput=off  SatLimitsSource=internal  UpperSaturationLimit=inf  LowerSaturationLimit=-inf  LinearizeAsGain=off  AntiWindupMode=none  Kb=1  POutMin=[]  POutMax=[]  IOutMin=[]  IOutMax=[]  DOutMin=[]  DOutMax=[]  NOutMin=[]  NOutMax=[]  SumOutMin=[]  SumOutMax=[]  SaturationOutMin=[]  SaturationOutMax=[]  PParamMin=[]  PParamMax=[]  IParamMin=[]  IParamMax=[]  DParamMin=[]  DParamMax=[]  NParamMin=[]  NParamMax=[]  KbParamMin=[]  KbParamMax=[]  KtParamMin=[]  KtParamMax=[]  KbOutMin=[]  KbOutMax=[]  KtOutMin=[]  KtOutMax=[]  IntegratorOutMin=[]  IntegratorOutMax=[]  FilterOutMin=[]  FilterOutMax=[]  SumI1OutMin=[]  SumI1OutMax=[]  SumI2OutMin=[]  SumI2OutMax=[]  SumI3OutMin=[]  SumI3OutMax=[]  SumI4OutMin=[]  SumI4OutMax=[]  SumDOutMin=[]  SumDOutMax=[]  DifferentiatorOutMin=[]  DifferentiatorOutMax=[]  FilterDiffOutCoefMin=[]  FilterDiffOutCoefMax=[]  ReciprocalOutMin=[]  ReciprocalOutMax=[]  SumDenOutMin=[]  SumDenOutMax=[]  SumNumOutMin=[]  SumNumOutMax=[]  DivideOutMin=[]  DivideOutMax=[]  UdiffTsProdOutMin=[]  UdiffTsProdOutMax=[]  NTsProdOutMin=[]  NTsProdOutMax=[]  UintegralTsProdOutMin=[]  UintegralTsProdOutMax=[]  UngainTsProdOutMin=[]  UngainTsProdOutMax=[]  IntegratorContinuousStateAttributes=''  IntegratorStateMustResolveToSignalObject=off  IntegratorRTWStateStorageClass=Auto  FilterContinuousStateAttributes=''  FilterStateMustResolveToSignalObject=off  FilterRTWStateStorageClass=Auto  ParallelPVariant=InternalParameters  IdealPVariant=Disabled  IVariant=InternalParameters  DVariant=InternalParameters  IntegratorVariant=Discrete  SatVariant=Disabled  AWVariant=Passthrough  PCopyVariant=Disabled  TRVariant=Disabled  FdbkBlocksVariant=Forward  IdealPFdbkVariant=Disabled  SatFdbkVariant=Disabled  DerivativeFilterVariant=ForwardEulerFilter  NVariant=InternalParameters  NCopyVariant=Disabled  FilterICVariant=InternalICsFilter  IntegratorICVariant=InternalICs  ExternalResetVariant=Disabled  TRSumVariant=Passthrough  SumFdbkVariant=Disabled  SumVariant=Sum_PID  TsampFilterVariant=InternalTs  TsampNgainVariant=Passthrough  TsampIntegralVariant=Passthrough  ExternalSaturationOutDataTypeStr=Inherit: Same as second input
  emi_377 : DiscreteFir
  emi_378 : Math  SaturateOnIntegerOverflow=on
  emi_379 : Product  Inputs=*
  emi_380 : Sin  TimeSource=Use external signal  SampleTime=0
  emi_381 : DiscreteIntegrator  SampleTime=-1  ICPrevOutput=DiscIntNeverNeededParam  ICPrevScaledInput=DiscIntNeverNeededParam
  emi_382 : DiscreteZeroPole  Poles=[0 0.5]  Gain=1  SampleTime=-1
  emi_383 : Abs
  emi_384 : Sum  Inputs=+
  emi_385 : simulink/Discrete/Transfer Fcn First Order  PoleZ=0.95  ICPrevOutput=0.0  DoSatur=off
  emi_386 : Sum  Inputs=+
  emi_387 : simulink/Discontinuities/Saturation Dynamic  OutMin=[]  OutMax=[]  OutDataTypeStr=Inherit: Same as second input  OutDataType=fixdt(1, 16)  OutScaling=2^-10  DoSatur=off
  emi_388 : simulink/Discrete/Transfer Fcn First Order  PoleZ=0.95  ICPrevOutput=0.0  DoSatur=off
  emi_389 : Math  SaturateOnIntegerOverflow=on
  emi_390 : Math  SaturateOnIntegerOverflow=on
  emi_391 : Product  Inputs=*
  emi_392 : simulink/Discontinuities/PWM  DisableCoverage=on  Period=1  DisallowZeroDutyCycle=off  RunAtFixedTimeIntervals=off  SampleTime=0.1
  emi_393 : Rounding
  emi_394 : DiscreteFir
  emi_395 : Trigonometry
  emi_396 : simulink/Discrete/Transfer Fcn First Order  PoleZ=0.95  ICPrevOutput=0.0  DoSatur=off
  emi_397 : simulink/Discrete/Difference  ICPrevInput=0.0  OutMin=[]  OutMax=[]  OutDataType=fixdt(1, 16)  OutScaling=2^-10  DoSatur=off
  emi_398 : Gain
  emi_399 : SignalGenerator  Units=rad/sec
  Out1 : Outport
  emi_365 : Outport  Port=2
  wires:
  In1/1 -> Out1/1
  emi_366/1 -> emi_367/1
  emi_367/1 -> emi_368/1
  emi_368/1 -> emi_369/1
  emi_369/1 -> emi_370/1
  emi_370/1 -> emi_371/1
  emi_371/1 -> emi_372/1
  emi_372/1 -> emi_373/1
  emi_373/1 -> emi_374/1
  emi_374/1 -> emi_375/1
  emi_375/1 -> emi_376/1
  emi_376/1 -> emi_377/1
  emi_377/1 -> emi_378/1
  emi_378/1 -> emi_379/1
  emi_379/1 -> emi_380/1
  emi_380/1 -> emi_381/1
  emi_381/1 -> emi_382/1
  emi_382/1 -> emi_383/1
  emi_383/1 -> emi_384/1
  emi_384/1 -> emi_385/1
  emi_385/1 -> emi_386/1
  emi_386/1 -> emi_387/1
  emi_387/1 -> emi_388/1
  emi_388/1 -> emi_389/1
  emi_389/1 -> emi_390/1
  emi_390/1 -> emi_391/1
  emi_391/1 -> emi_392/1
  emi_392/1 -> emi_393/1
  emi_393/1 -> emi_394/1
  emi_394/1 -> emi_395/1
  emi_395/1 -> emi_396/1
  emi_396/1 -> emi_397/1
  emi_397/1 -> emi_398/1
  emi_399/1 -> emi_366/1
  emi_398/1 -> emi_365/1

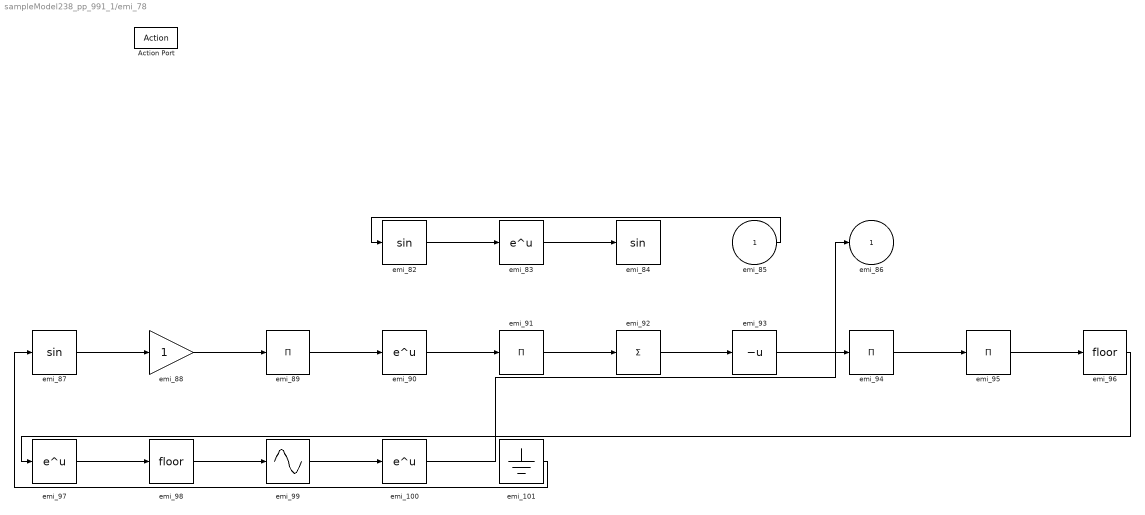
== system sampleModel238_pp_991_1/emi_78 ==
  emi_85 : Inport
  Action Port : ActionPort  ActionPortLabel=if(0 > u1)
  emi_100 : Math  SaturateOnIntegerOverflow=on
  emi_101 : Ground
  emi_82 : Trigonometry  SampleTime=1
  emi_83 : Math  SampleTime=1  SaturateOnIntegerOverflow=on
  emi_84 : Trigonometry  SampleTime=1
  emi_87 : Trigonometry
  emi_88 : Gain
  emi_{89,91,94..95} (4 alike) : Product  Inputs=*
  emi_90 : Math  SaturateOnIntegerOverflow=on
  emi_92 : Sum  Inputs=+
  emi_93 : UnaryMinus
  emi_96 : Rounding
  emi_97 : Math  SaturateOnIntegerOverflow=on
  emi_98 : Rounding
  emi_99 : Sin  TimeSource=Use external signal  SampleTime=0
  emi_86 : Outport
  wires:
  emi_85/1 -> emi_82/1
  emi_82/1 -> emi_83/1
  emi_83/1 -> emi_84/1
  emi_87/1 -> emi_88/1
  emi_88/1 -> emi_89/1
  emi_89/1 -> emi_90/1
  emi_90/1 -> emi_91/1
  emi_91/1 -> emi_92/1
  emi_92/1 -> emi_93/1
  emi_93/1 -> emi_94/1
  emi_94/1 -> emi_95/1
  emi_95/1 -> emi_96/1
  emi_96/1 -> emi_97/1
  emi_97/1 -> emi_98/1
  emi_98/1 -> emi_99/1
  emi_99/1 -> emi_100/1
  emi_101/1 -> emi_87/1
  emi_100/1 -> emi_86/1
